simulink model "gm_sampleModel1668_sub"  (R2023a)
settings: Solver=VariableStepAuto  StartTime=0.0  StopTime=10.0  RelTol=1e-3
libraries: hdlsllib x2, simulink x1
settings Model: Creator=user1  LastModifiedBy=user1
settings OptimizationCC: BlockReduction=off  ConditionallyExecuteInputs=off
settings DebuggingCC: InheritedTsInSrcMsg=none

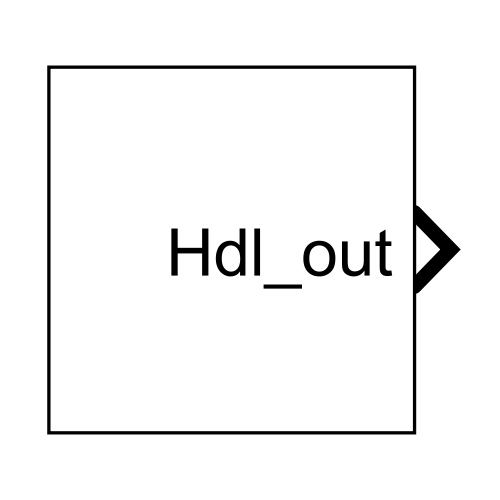
[thumbnail: Simulink's stored preview of the top-level diagram]
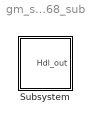
== system gm_sampleModel1668_sub ==
  Subsystem : Subsystem

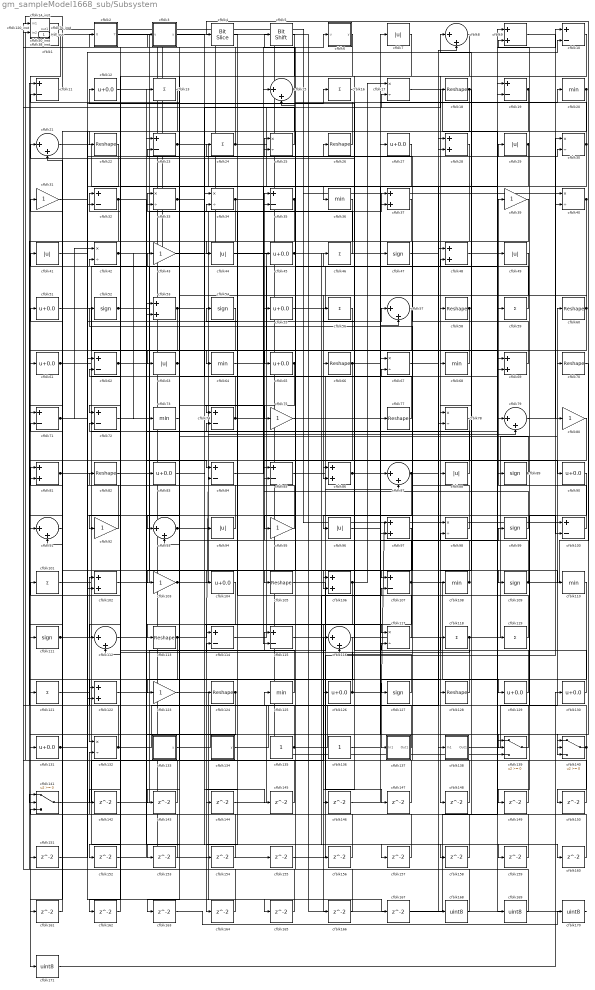
== system gm_sampleModel1668_sub/Subsystem ==
  cfblk1 : simulink/Logic and Bit Operations/Bit Set  iBit=0
      settings: LibrarySourceBlock=|
      | hdlsllib/Logic and Bit
      | Operations/Bit Set
  cfblk{10..11,19,23,32,35,62,71..72,74,84..85,100,107,114..115} (16 alike) : Sum  Inputs=+-  OutDataTypeStr=uint8
  cfblk{13,16,24,46,56,59,101,118..119,121} (10 alike) : Sum  Inputs=+  OutDataTypeStr=uint8
  cfblk{9,28,37,48,53,69,81,86,97,102,106,122} (12 alike) : Sum  OutDataTypeStr=uint8
  cfblk{31,39,43,75,80,92,95,103,123} (9 alike) : Gain  OutDataTypeStr=uint8
  cfblk{12,27,45,51,55,61,65,83,90,104,126,129..131} (14 alike) : Bias  Bias=0.0  SaturateOnIntegerOverflow=off
  cfblk{18,22,26,58,60,66,70,77,82,105,113,124,128} (13 alike) : Reshape
  cfblk{20,36,64,68,73,108,110,125} (8 alike) : MinMax  OutDataTypeStr=uint8
  cfblk{47,52,54,89,99,109,111,127} (8 alike) : Signum
  cfblk{8,15,21,57,79,87,91,93,112,116} (10 alike) : Sum  Inputs=|++  OutDataTypeStr=uint8
  cfblk{17,25,30,33..34,40,42,67,78,98,117,132} (12 alike) : Product  Inputs=*/  OutDataTypeStr=uint8  RndMeth=Zero  SaturateOnIntegerOverflow=on
  cfblk120_inst : Subsystem
  cfblk133 : Subsystem  mask(Counter Free-Running){NumBits=double(16), tsamp=double(-1)}
      mask prompts: NumBits "Simulink:masks:NumberOfBits_MP"; tsamp "Simulink:masks:SampleTime_MP"
      mask help: Simulink:masks:CounterFreeRunning_MD
  cfblk134 : Subsystem  mask(Counter Free-Running){NumBits=double(16), tsamp=double(-1)}
      mask prompts: NumBits "Simulink:masks:NumberOfBits_MP"; tsamp "Simulink:masks:SampleTime_MP"
      mask help: Simulink:masks:CounterFreeRunning_MD
  cfblk135 : Constant  OutDataTypeStr=uint8  SampleTime=-1
  cfblk136 : Constant  OutDataTypeStr=uint8  SampleTime=-1
  cfblk137 : Subsystem
  cfblk138 : Subsystem
  cfblk139 : Switch  OutDataTypeStr=uint8  SaturateOnIntegerOverflow=off  InputSameDT=off
  cfblk140 : Switch  OutDataTypeStr=uint8  SaturateOnIntegerOverflow=off  InputSameDT=off
  cfblk141 : Switch  OutDataTypeStr=uint8  SaturateOnIntegerOverflow=off  InputSameDT=off
  cfblk{142..167} (26 alike) : Delay  SampleTime=1
  cfblk14_inst : Subsystem
  cfblk{168..171} (4 alike) : DataTypeConversion  OutDataTypeStr=uint8  SaturateOnIntegerOverflow=off  RndMeth=Floor
  cfblk2 : Subsystem  mask(Detect Rise Nonnegative){vinit=double(0), InputProcessing=Elements as channels (sample based), OutDataTypeStr=uint8}
      mask prompts: vinit "Simulink:masks:InitialCondition_MP"; InputProcessing "Simulink:masks:InputProcessing_MP"; OutDataTypeStr "Simulink:masks:OutputDataType_MP"
      mask help: Simulink:masks:DetectRiseNonnegative_MD
      mask init:
      | InputProcessing = 'Elements as channels (sample based)';
      | OutDataTypeStr = 'uint8';
      | vinit = double(0);
      mask TypeOptions InputProcessing: Simulink:masks:ColumnsAsChannelsFrameBased | Simulink:masks:ElementsAsChannelsSampleBased
      mask TypeOptions OutDataTypeStr: Simulink:masks:uint8 | Simulink:masks:boolean
      mask Display: fprintf('U >= 0\n&  NOT\nU/z >= 0')
  cfblk{7,29,41,44,49,63,88,94,96} (9 alike) : Abs  OutDataTypeStr=uint8  SaturateOnIntegerOverflow=off
  cfblk3 : Subsystem  mask(Compare To Constant){relop=<=, const=double(3), OutDataTypeStr=uint8, ZeroCross=on}
      mask prompts: relop "Simulink:masks:Operator_MP"; const "Simulink:masks:ConstantValue_MP"; OutDataTypeStr "Simulink:masks:OutputDataType_MP"; ZeroCross "Simulink:masks:EnableZerocrossingDetection_MP"
      mask help: Simulink:masks:CompareToConstant_MD
      mask init:
      | OutDataTypeStr = 'uint8';
      | ZeroCross = 'on';
      | blkName = 'sampleModel1668_sub/Subsystem/cfblk3';
      | const = double(3);
      | const_str = '3.0';
      | const_val = double(3);
      | relop = '<=';
      | setValue = 'fixdt(0, 8)';
      | str = '<= 3';
      mask TypeOptions relop: == | ~= | < | <= | >= | >
      mask TypeOptions OutDataTypeStr: Simulink:masks:uint8 | Simulink:masks:boolean
      mask Callback ZeroCross: sl('zeroCrossEnable', gcbh);
      mask Display: disp(str)
  cfblk38_inst : Subsystem
  cfblk4 : hdlsllib/Logic and Bit Operations/Bit Slice  lidx=7  ridx=0
  cfblk5 : hdlsllib/Logic and Bit Operations/Bit Shift  mode=Shift Left Logical  N=0
  cfblk50_inst : Subsystem
  cfblk6 : Subsystem  mask(Compare To Constant){relop=<=, const=double(3), OutDataTypeStr=uint8, ZeroCross=on}
      mask prompts: relop "Simulink:masks:Operator_MP"; const "Simulink:masks:ConstantValue_MP"; OutDataTypeStr "Simulink:masks:OutputDataType_MP"; ZeroCross "Simulink:masks:EnableZerocrossingDetection_MP"
      mask help: Simulink:masks:CompareToConstant_MD
      mask init:
      | OutDataTypeStr = 'uint8';
      | ZeroCross = 'on';
      | blkName = 'sampleModel1668_sub/Subsystem/cfblk6';
      | const = double(3);
      | const_str = '3.0';
      | const_val = double(3);
      | relop = '<=';
      | setValue = 'fixdt(0, 8)';
      | str = '<= 3';
      mask TypeOptions relop: == | ~= | < | <= | >= | >
      mask TypeOptions OutDataTypeStr: Simulink:masks:uint8 | Simulink:masks:boolean
      mask Callback ZeroCross: sl('zeroCrossEnable', gcbh);
      mask Display: disp(str)
  cfblk76_inst : Subsystem
  Hdl_out : Outport  OutDataTypeStr=uint8  SampleTime=1
  wires:
  cfblk1/1 -> cfblk171/1
  cfblk10/1 -> cfblk148/1
  cfblk100/1 -> cfblk39/1
  cfblk101/1 -> cfblk69/1
  cfblk102/1 -> cfblk46/1
  cfblk103/1 -> cfblk79/2, cfblk37/1
  cfblk104/1 -> cfblk164/1
  cfblk105/1 -> cfblk147/1
  cfblk106/1 -> cfblk113/1, cfblk17/1
  cfblk107/1 -> cfblk35/1, cfblk129/1, cfblk166/1
  cfblk108/1 -> cfblk41/1, cfblk98/2
  cfblk109/1 -> cfblk4/1, cfblk11/2
  cfblk11/1 -> cfblk38_inst/1(in1)
  cfblk110/1 -> cfblk137/1(In1)
  cfblk111/1 -> cfblk49/1, cfblk157/1
  cfblk112/1 -> cfblk128/1
  cfblk113/1 -> cfblk84/2, cfblk121/1
  cfblk114/1 -> cfblk48/2
  cfblk115/1 -> cfblk79/1
  cfblk116/1 -> cfblk132/1
  cfblk117/1 -> cfblk34/2
  cfblk118/1 -> cfblk60/1, cfblk114/2
  cfblk119/1 -> cfblk54/1
  cfblk12/1 -> cfblk104/1
  cfblk120_inst/1(out1) -> cfblk40/1
  cfblk121/1 -> cfblk102/1
  cfblk122/1 -> cfblk87/2
  cfblk123/1 -> cfblk167/1
  cfblk124/1 -> cfblk152/1, cfblk151/1
  cfblk125/1 -> cfblk101/1
  cfblk126/1 -> cfblk97/1, cfblk42/2
  cfblk127/1 -> cfblk116/2
  cfblk128/1 -> cfblk12/1
  cfblk129/1 -> cfblk21/1
  cfblk13/1 -> cfblk131/1
  cfblk130/1 -> cfblk118/1
  cfblk131/1 -> cfblk57/1, cfblk16/1
  cfblk132/1 -> cfblk8/2, cfblk11/1
  cfblk133/1(y) -> cfblk125/1
  cfblk134/1(y) -> cfblk67/1
  cfblk135/1 -> cfblk77/1, cfblk72/2, cfblk50_inst/1(in1)
  cfblk136/1 -> cfblk99/1
  cfblk137/1(Out1) -> cfblk21/2
  cfblk138/1(Out1) -> cfblk70/1
  cfblk139/1 -> cfblk67/2
  cfblk14_inst/1(out1) -> cfblk139/3, cfblk100/1
  cfblk140/1 -> cfblk9/2, cfblk9/1, cfblk150/1
  cfblk141/1 -> cfblk116/1
  cfblk142/1 -> cfblk107/2
  cfblk143/1 -> cfblk14_inst/1(in1)
  cfblk144/1 -> cfblk28/2
  cfblk145/1 -> cfblk33/1
  cfblk146/1 -> cfblk87/1
  cfblk147/1 -> cfblk71/2
  cfblk148/1 -> cfblk117/2
  cfblk149/1 -> cfblk120_inst/2(in2)
  cfblk15/1 -> cfblk76_inst/1(in1), cfblk72/1
  cfblk150/1 -> cfblk81/1
  cfblk151/1 -> cfblk30/2
  cfblk152/1 -> cfblk53/2
  cfblk153/1 -> cfblk62/2
  cfblk154/1 -> cfblk32/1
  cfblk155/1 -> cfblk40/2
  cfblk156/1 -> cfblk35/2
  cfblk157/1 -> cfblk115/1
  cfblk158/1 -> cfblk141/3
  cfblk159/1 -> cfblk8/1
  cfblk16/1 -> cfblk146/1
  cfblk160/1 -> cfblk132/2
  cfblk161/1 -> cfblk91/2
  cfblk162/1 -> cfblk122/1
  cfblk163/1 -> cfblk170/1
  cfblk164/1 -> cfblk141/1
  cfblk165/1 -> cfblk76_inst/2(in2)
  cfblk166/1 -> cfblk15/2
  cfblk167/1 -> cfblk19/2
  cfblk168/1 -> cfblk51/1
  cfblk169/1 -> cfblk2/1(U)
  cfblk17/1 -> cfblk59/1
  cfblk170/1 -> cfblk1/1
  cfblk171/1 -> cfblk130/1
  cfblk18/1 -> cfblk102/2, cfblk78/1
  cfblk19/1 -> cfblk71/1, cfblk108/1
  cfblk2/1(Y) -> cfblk168/1
  cfblk20/1 -> cfblk74/1, cfblk65/1
  cfblk21/1 -> cfblk36/1
  cfblk22/1 -> cfblk32/2
  cfblk23/1 -> cfblk97/2, cfblk85/1
  cfblk24/1 -> cfblk89/1, cfblk18/1, cfblk14_inst/2(in2), cfblk127/1
  cfblk25/1 -> cfblk38_inst/2(in2)
  cfblk26/1 -> cfblk120_inst/1(in1)
  cfblk27/1 -> cfblk95/1
  cfblk28/1 -> cfblk44/1
  cfblk29/1 -> cfblk115/2, cfblk142/1
  cfblk3/1(y) -> cfblk109/1
  cfblk30/1 -> cfblk50_inst/2(in2), cfblk144/1, cfblk68/1
  cfblk31/1 -> cfblk26/1
  cfblk32/1 -> cfblk83/1, cfblk81/2
  cfblk33/1 -> cfblk75/1, cfblk117/1
  cfblk34/1 -> cfblk88/1, cfblk161/1
  cfblk35/1 -> cfblk91/1, cfblk112/2
  cfblk36/1 -> cfblk114/1
  cfblk37/1 -> cfblk162/1
  cfblk38_inst/1(out1) -> cfblk155/1
  cfblk39/1 -> cfblk107/1
  cfblk4/1 -> cfblk154/1
  cfblk40/1 -> cfblk86/2, cfblk106/2, cfblk78/2
  cfblk41/1 -> cfblk100/2
  cfblk42/1 -> cfblk15/1, cfblk73/1
  cfblk43/1 -> cfblk94/1
  cfblk44/1 -> cfblk69/2
  cfblk45/1 -> cfblk140/3, cfblk159/1, Hdl_out/1
  cfblk46/1 -> cfblk33/2
  cfblk47/1 -> cfblk28/1
  cfblk48/1 -> cfblk169/1
  cfblk49/1 -> cfblk63/1
  cfblk5/1 -> cfblk112/1
  cfblk50_inst/1(out1) -> cfblk119/1
  cfblk51/1 -> cfblk138/1(In1)
  cfblk52/1 -> cfblk45/1, cfblk139/2
  cfblk53/1 -> cfblk98/1, cfblk92/1, cfblk17/2
  cfblk54/1 -> cfblk143/1
  cfblk55/1 -> cfblk7/1
  cfblk56/1 -> cfblk61/1
  cfblk57/1 -> cfblk105/1
  cfblk58/1 -> cfblk96/1, cfblk126/1
  cfblk59/1 -> cfblk25/1
  cfblk6/1(y) -> cfblk22/1
  cfblk60/1 -> cfblk93/1, cfblk58/1
  cfblk61/1 -> cfblk48/1, cfblk165/1
  cfblk62/1 -> cfblk29/1, cfblk25/2, cfblk158/1
  cfblk63/1 -> cfblk93/2, cfblk153/1
  cfblk64/1 -> cfblk6/1(u)
  cfblk65/1 -> cfblk5/1, cfblk163/1
  cfblk66/1 -> cfblk139/1, cfblk122/2
  cfblk67/1 -> cfblk160/1
  cfblk68/1 -> cfblk64/1
  cfblk69/1 -> cfblk24/1
  cfblk7/1 -> cfblk103/1
  cfblk70/1 -> cfblk140/2
  cfblk71/1 -> cfblk10/2, cfblk42/1
  cfblk72/1 -> cfblk84/1
  cfblk73/1 -> cfblk123/1
  cfblk74/1 -> cfblk90/1, cfblk43/1
  cfblk75/1 -> cfblk140/1
  cfblk76_inst/1(out1) -> cfblk47/1
  cfblk77/1 -> cfblk34/1
  cfblk78/1 -> cfblk141/2
  cfblk79/1 -> cfblk30/1
  cfblk8/1 -> cfblk66/1
  cfblk80/1 -> cfblk124/1
  cfblk81/1 -> cfblk74/2, cfblk57/2, cfblk10/1, cfblk13/1
  cfblk82/1 -> cfblk110/1
  cfblk83/1 -> cfblk145/1
  cfblk84/1 -> cfblk55/1
  cfblk85/1 -> cfblk27/1
  cfblk86/1 -> cfblk37/2, cfblk56/1
  cfblk87/1 -> cfblk106/1, cfblk20/1
  cfblk88/1 -> cfblk53/1
  cfblk89/1 -> cfblk86/1, cfblk23/2
  cfblk9/1 -> cfblk80/1
  cfblk90/1 -> cfblk149/1
  cfblk91/1 -> cfblk31/1
  cfblk92/1 -> cfblk62/1
  cfblk93/1 -> cfblk156/1, cfblk3/1(u)
  cfblk94/1 -> cfblk23/1
  cfblk95/1 -> cfblk82/1
  cfblk96/1 -> cfblk19/1
  cfblk97/1 -> cfblk111/1
  cfblk98/1 -> cfblk52/1
  cfblk99/1 -> cfblk85/2

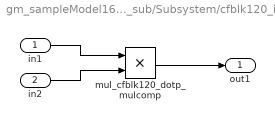
== system gm_sampleModel1668_sub/Subsystem/cfblk120_inst ==
  in1 : Inport  OutDataTypeStr=uint8  SampleTime=1
  in2 : Inport  Port=2  OutDataTypeStr=uint8  SampleTime=1
  mul_cfblk120_dotp_mulcomp : Product  Inputs=**  OutDataTypeStr=uint8  SampleTime=1
  out1 : Outport  OutDataTypeStr=uint8  SampleTime=1
  wires:
  in1/1 -> mul_cfblk120_dotp_mulcomp/1
  in2/1 -> mul_cfblk120_dotp_mulcomp/2
  mul_cfblk120_dotp_mulcomp/1 -> out1/1

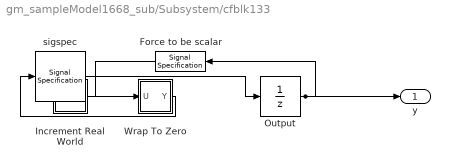
== system gm_sampleModel1668_sub/Subsystem/cfblk133 ==
  Force to be scalar : SignalSpecification  DisableCoverage=on  Dimensions=1
  Increment Real World : Subsystem  mask(Real World Value Increment){}
      mask help: Simulink:masks:RealWorldValueIncrement_MD
      mask Display: disp('V++')
  Output : UnitDelay  InitialCondition=0.0  SampleTime=tsamp  HasFrameUpgradeWarning=on
  Wrap To Zero : Subsystem  mask(Wrap To Zero){Threshold=double(65535)}
      mask prompts: Threshold "Simulink:masks:Threshold_MP"
      mask help: Simulink:masks:WrapToZero_MD
  sigspec : SignalSpecification  OutDataTypeStr=uint16  Dimensions=1
  y : Outport  SampleTime=1
  wires:
  Force to be scalar/1 -> Increment Real World/1(u)
  Increment Real World/1(y) -> Wrap To Zero/1(U)
  Output/1 -> Force to be scalar/1, y/1
  Wrap To Zero/1(Y) -> sigspec/1
  sigspec/1 -> Output/1

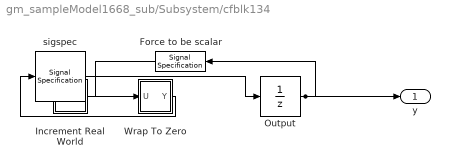
== system gm_sampleModel1668_sub/Subsystem/cfblk134 ==
  Force to be scalar : SignalSpecification  DisableCoverage=on  Dimensions=1
  Increment Real World : Subsystem  mask(Real World Value Increment){}
      mask help: Simulink:masks:RealWorldValueIncrement_MD
      mask Display: disp('V++')
  Output : UnitDelay  InitialCondition=0.0  SampleTime=tsamp  HasFrameUpgradeWarning=on
  Wrap To Zero : Subsystem  mask(Wrap To Zero){Threshold=double(65535)}
      mask prompts: Threshold "Simulink:masks:Threshold_MP"
      mask help: Simulink:masks:WrapToZero_MD
  sigspec : SignalSpecification  OutDataTypeStr=uint16  Dimensions=1
  y : Outport  SampleTime=1
  wires:
  Force to be scalar/1 -> Increment Real World/1(u)
  Increment Real World/1(y) -> Wrap To Zero/1(U)
  Output/1 -> Force to be scalar/1, y/1
  Wrap To Zero/1(Y) -> sigspec/1
  sigspec/1 -> Output/1

== system gm_sampleModel1668_sub/Subsystem/cfblk137 ==
  In1 : Inport  OutDataTypeStr=uint8  PortDimensions=1  SampleTime=1
  Out1 : Outport  SampleTime=1
  wires:
  In1/1 -> Out1/1

== system gm_sampleModel1668_sub/Subsystem/cfblk138 ==
  In1 : Inport  OutDataTypeStr=uint8  PortDimensions=1  SampleTime=1
  Out1 : Outport  SampleTime=1
  wires:
  In1/1 -> Out1/1

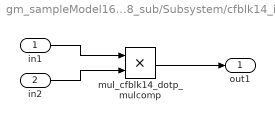
== system gm_sampleModel1668_sub/Subsystem/cfblk14_inst ==
  in1 : Inport  OutDataTypeStr=uint8  SampleTime=1
  in2 : Inport  Port=2  OutDataTypeStr=uint8  SampleTime=1
  mul_cfblk14_dotp_mulcomp : Product  Inputs=**  OutDataTypeStr=uint8  SampleTime=1
  out1 : Outport  OutDataTypeStr=uint8  SampleTime=1
  wires:
  in1/1 -> mul_cfblk14_dotp_mulcomp/1
  in2/1 -> mul_cfblk14_dotp_mulcomp/2
  mul_cfblk14_dotp_mulcomp/1 -> out1/1

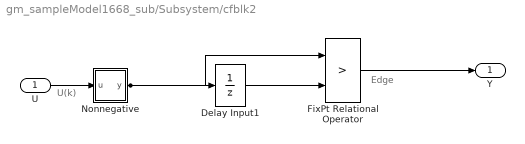
== system gm_sampleModel1668_sub/Subsystem/cfblk2 ==
  note: U(k)
  note: Edge
  U : Inport  OutDataTypeStr=uint8  SampleTime=1
  Delay Input1 : UnitDelay  Description=Store in Global RAM  DisableCoverage=on  InitialCondition=vinit  SampleTime=-1  HasFrameUpgradeWarning=on
  FixPt Relational Operator : RelationalOperator  Operator=>  OutDataTypeStr=fixdt(0, 8)  ZeroCross=off  InputSameDT=off
  Nonnegative : Subsystem  mask(Compare To Zero){relop=>=, OutDataTypeStr=boolean, ZeroCross=off}
      mask prompts: relop "Simulink:masks:Operator_MP"; OutDataTypeStr "Simulink:masks:OutputDataType_MP"; ZeroCross "Simulink:masks:EnableZerocrossingDetection_MP"
      mask help: Simulink:masks:CompareToZero_MD
      mask init:
      | OutDataTypeStr = 'boolean';
      | ZeroCross = 'off';
      | blkName = 'sampleModel1668_sub/Subsystem/cfblk2/Nonnegative';
      | relop = '>=';
      | setValue = 'boolean';
      mask TypeOptions relop: == | ~= | < | <= | >= | >
      mask TypeOptions OutDataTypeStr: Simulink:masks:uint8 | Simulink:masks:boolean
      mask Callback ZeroCross: sl('zeroCrossEnable', gcbh);
      mask Display: disp([relop,' 0'])
  Y : Outport  SampleTime=1
  wires:
  U/1 -> Nonnegative/1(u)
  Delay Input1/1 -> FixPt Relational Operator/2
  FixPt Relational Operator/1 -> Y/1
  Nonnegative/1(y) -> FixPt Relational Operator/1, Delay Input1/1

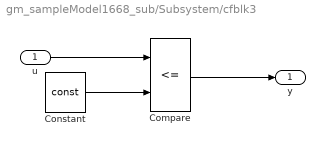
== system gm_sampleModel1668_sub/Subsystem/cfblk3 ==
  u : Inport  OutDataTypeStr=uint8  SampleTime=1
  Compare : RelationalOperator  Operator=<=  OutDataTypeStr=fixdt(0, 8)
  Constant : Constant  DisableCoverage=on  Value=const  OutDataTypeStr=Inherit: Inherit via back propagation  SampleTime=-1
  y : Outport  SampleTime=1
  wires:
  u/1 -> Compare/1
  Compare/1 -> y/1
  Constant/1 -> Compare/2

== system gm_sampleModel1668_sub/Subsystem/cfblk38_inst ==
  in1 : Inport  OutDataTypeStr=uint8  SampleTime=1
  in2 : Inport  Port=2  OutDataTypeStr=uint8  SampleTime=1
  mul_cfblk38_dotp_mulcomp : Product  Inputs=**  OutDataTypeStr=uint8  SampleTime=1
  out1 : Outport  OutDataTypeStr=uint8  SampleTime=1
  wires:
  in1/1 -> mul_cfblk38_dotp_mulcomp/1
  in2/1 -> mul_cfblk38_dotp_mulcomp/2
  mul_cfblk38_dotp_mulcomp/1 -> out1/1

== system gm_sampleModel1668_sub/Subsystem/cfblk50_inst ==
  in1 : Inport  OutDataTypeStr=uint8  SampleTime=1
  in2 : Inport  Port=2  OutDataTypeStr=uint8  SampleTime=1
  mul_cfblk50_dotp_mulcomp : Product  Inputs=**  OutDataTypeStr=uint8  SampleTime=1
  out1 : Outport  OutDataTypeStr=uint8  SampleTime=1
  wires:
  in1/1 -> mul_cfblk50_dotp_mulcomp/1
  in2/1 -> mul_cfblk50_dotp_mulcomp/2
  mul_cfblk50_dotp_mulcomp/1 -> out1/1

== system gm_sampleModel1668_sub/Subsystem/cfblk6 ==
  u : Inport  OutDataTypeStr=uint8  SampleTime=1
  Compare : RelationalOperator  Operator=<=  OutDataTypeStr=fixdt(0, 8)
  Constant : Constant  DisableCoverage=on  Value=const  OutDataTypeStr=Inherit: Inherit via back propagation  SampleTime=-1
  y : Outport  SampleTime=1
  wires:
  u/1 -> Compare/1
  Compare/1 -> y/1
  Constant/1 -> Compare/2

== system gm_sampleModel1668_sub/Subsystem/cfblk76_inst ==
  in1 : Inport  OutDataTypeStr=uint8  SampleTime=1
  in2 : Inport  Port=2  OutDataTypeStr=uint8  SampleTime=1
  mul_cfblk76_dotp_mulcomp : Product  Inputs=**  OutDataTypeStr=uint8  SampleTime=1
  out1 : Outport  OutDataTypeStr=uint8  SampleTime=1
  wires:
  in1/1 -> mul_cfblk76_dotp_mulcomp/1
  in2/1 -> mul_cfblk76_dotp_mulcomp/2
  mul_cfblk76_dotp_mulcomp/1 -> out1/1

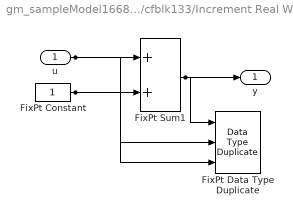
== system gm_sampleModel1668_sub/Subsystem/cfblk133/Increment Real World ==
  u : Inport  OutDataTypeStr=uint16  SampleTime=1
  FixPt Constant : Constant  DisableCoverage=on  OutDataTypeStr=Inherit: Inherit via back propagation  SampleTime=-1
  FixPt Data Type Duplicate : DataTypeDuplicate  DisableCoverage=on  NumInputPorts=3
  FixPt Sum1 : Sum  InputSameDT=on  OutDataTypeStr=Inherit: Inherit via back propagation  LockScale=on
  y : Outport  SampleTime=1
  wires:
  u/1 -> FixPt Sum1/1, FixPt Data Type Duplicate/2
  FixPt Constant/1 -> FixPt Sum1/2, FixPt Data Type Duplicate/3
  FixPt Sum1/1 -> FixPt Data Type Duplicate/1, y/1

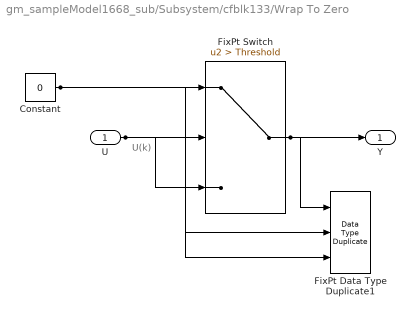
== system gm_sampleModel1668_sub/Subsystem/cfblk133/Wrap To Zero ==
  note: U(k)
  U : Inport  OutDataTypeStr=uint16  SampleTime=1
  Constant : Constant  DisableCoverage=on  Value=0  OutDataTypeStr=Inherit: Inherit via back propagation  SampleTime=-1
  FixPt Data Type Duplicate1 : DataTypeDuplicate  DisableCoverage=on  NumInputPorts=3
  FixPt Switch : Switch  Criteria=u2 > Threshold  Threshold=Threshold  OutDataTypeStr=Inherit: Inherit via back propagation  ZeroCross=off  SaturateOnIntegerOverflow=off  InputSameDT=off
  Y : Outport  SampleTime=1
  wires:
  U/1 -> FixPt Switch/3, FixPt Switch/2, FixPt Data Type Duplicate1/2
  Constant/1 -> FixPt Switch/1, FixPt Data Type Duplicate1/3
  FixPt Switch/1 -> FixPt Data Type Duplicate1/1, Y/1

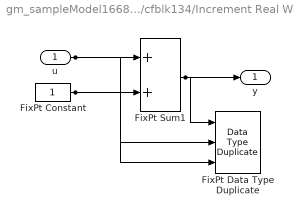
== system gm_sampleModel1668_sub/Subsystem/cfblk134/Increment Real World ==
  u : Inport  OutDataTypeStr=uint16  SampleTime=1
  FixPt Constant : Constant  DisableCoverage=on  OutDataTypeStr=Inherit: Inherit via back propagation  SampleTime=-1
  FixPt Data Type Duplicate : DataTypeDuplicate  DisableCoverage=on  NumInputPorts=3
  FixPt Sum1 : Sum  InputSameDT=on  OutDataTypeStr=Inherit: Inherit via back propagation  LockScale=on
  y : Outport  SampleTime=1
  wires:
  u/1 -> FixPt Sum1/1, FixPt Data Type Duplicate/2
  FixPt Constant/1 -> FixPt Sum1/2, FixPt Data Type Duplicate/3
  FixPt Sum1/1 -> FixPt Data Type Duplicate/1, y/1

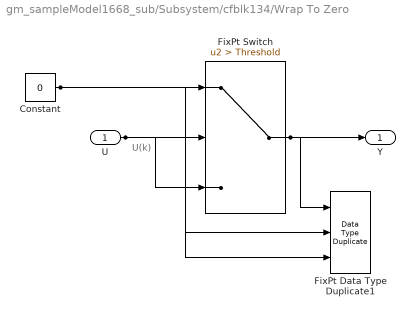
== system gm_sampleModel1668_sub/Subsystem/cfblk134/Wrap To Zero ==
  note: U(k)
  U : Inport  OutDataTypeStr=uint16  SampleTime=1
  Constant : Constant  DisableCoverage=on  Value=0  OutDataTypeStr=Inherit: Inherit via back propagation  SampleTime=-1
  FixPt Data Type Duplicate1 : DataTypeDuplicate  DisableCoverage=on  NumInputPorts=3
  FixPt Switch : Switch  Criteria=u2 > Threshold  Threshold=Threshold  OutDataTypeStr=Inherit: Inherit via back propagation  ZeroCross=off  SaturateOnIntegerOverflow=off  InputSameDT=off
  Y : Outport  SampleTime=1
  wires:
  U/1 -> FixPt Switch/3, FixPt Switch/2, FixPt Data Type Duplicate1/2
  Constant/1 -> FixPt Switch/1, FixPt Data Type Duplicate1/3
  FixPt Switch/1 -> FixPt Data Type Duplicate1/1, Y/1

== system gm_sampleModel1668_sub/Subsystem/cfblk2/Nonnegative ==
  u : Inport  OutDataTypeStr=uint8  SampleTime=1
  Compare : RelationalOperator  OutDataTypeStr=boolean  ZeroCross=off
  Constant : Constant  DisableCoverage=on  Value=0  OutDataTypeStr=Inherit: Inherit via back propagation  SampleTime=-1  PreserveConstantTs=on
  y : Outport  SampleTime=1
  wires:
  u/1 -> Compare/1
  Compare/1 -> y/1
  Constant/1 -> Compare/2
